simulink model "Q11_Simulation"  (R2022b)
settings: Solver=VariableStepAuto  StartTime=0.0  StopTime=10  RelTol=1e-3
undefined symbols (not defined in the file): A, B, C, L
settings Model: Creator=amirz  LastModifiedBy=amirz

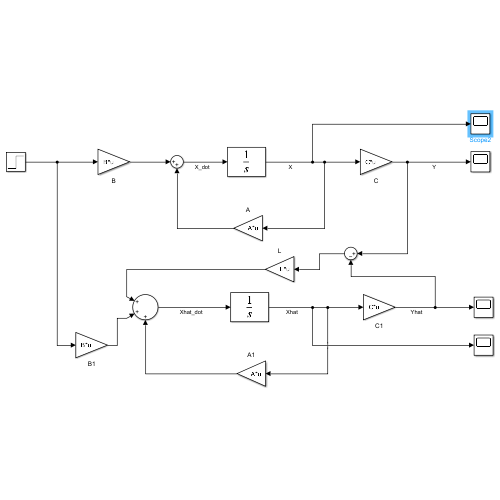
[thumbnail: Simulink's stored preview of the top-level diagram]
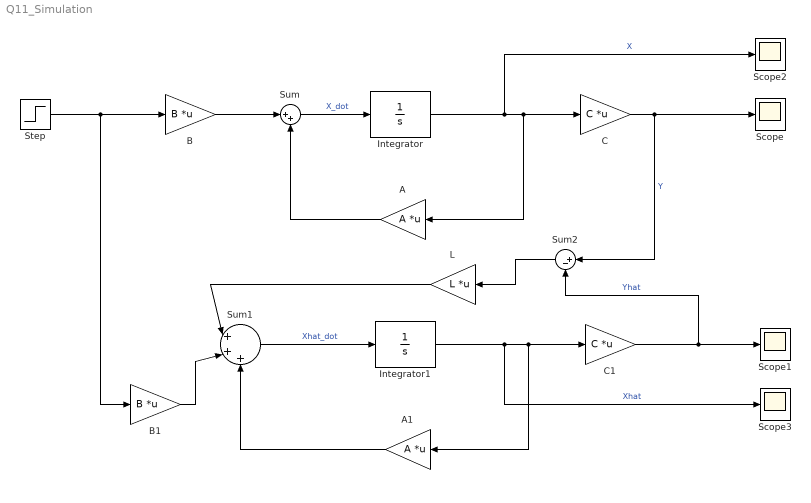
== system Q11_Simulation ==
  A : Gain  Gain=A  Multiplication=Matrix(K*u)
  A1 : Gain  Gain=A  Multiplication=Matrix(K*u)
  B : Gain  Gain=B  Multiplication=Matrix(K*u)
  B1 : Gain  Gain=B  Multiplication=Matrix(K*u)
  C : Gain  Gain=C  Multiplication=Matrix(K*u)
  C1 : Gain  Gain=C  Multiplication=Matrix(K*u)
  Integrator : Integrator
  Integrator1 : Integrator
  L : Gain  Gain=L  Multiplication=Matrix(K*u)
  Scope{,1..3} (4 alike) : Scope
  Step : Step  SampleTime=0
  Sum : Sum  Inputs=|++
  Sum1 : Sum  Inputs=|+++
  Sum2 : Sum  Inputs=|+-
  wires:
  C/1 -> Sum2/1, Scope/1  "Y"
  Step/1 -> B1/1, B/1
  Integrator/1 -> Scope2/1, A/1, C/1  "X"
  Sum/1 -> Integrator/1  "X_dot"
  A/1 -> Sum/2
  B/1 -> Sum/1
  C1/1 -> Scope1/1, Sum2/2  "Yhat"
  Integrator1/1 -> A1/1, C1/1, Scope3/1  "Xhat"
  Sum1/1 -> Integrator1/1  "Xhat_dot"
  Sum2/1 -> L/1
  L/1 -> Sum1/1
  A1/1 -> Sum1/3
  B1/1 -> Sum1/2
